simulink model "MirrorSubsystemrepo"  (R2018a)
settings: Solver=VariableStepAuto  StartTime=0.0  StopTime=10.0  RelTol=1e-3
undefined symbols (not defined in the file): sigbuilder_block
libraries: simulink x4
settings Model: Creator=Sushma  LastModifiedBy=training
settings DataIOCC: ReturnWorkspaceOutputs=on
settings SFSimCC: SimUseLocalCustomCode=on
settings RTWCC: RTWUseLocalCustomCode=on

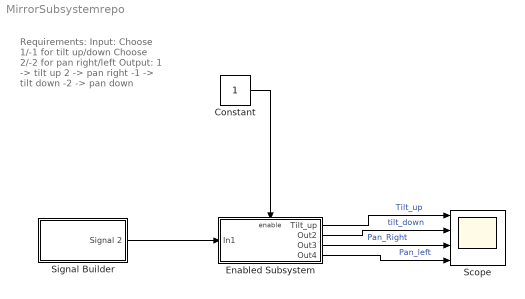
== system MirrorSubsystemrepo ==
  note: Requirements:
      | Input:
      | Choose 1/-1 for tilt up/down
      | Choose 2/-2 for pan right/left
      | Output:
      | 1  ->  tilt up
      | 2  -> pan right
      | -1 -> tilt down
      | -2 -> pan down
  Constant : Constant
  Enabled Subsystem : Subsystem  TreatAsAtomicUnit=on
  Scope : Scope  NumInputPorts=4
  Signal Builder : Subsystem  Tag=STV Subsys  LoadFcn=sigbuilder_block('load');  StartFcn=sigbuilder_block('start');  StopFcn=sigbuilder_block('stop');  ClipboardFcn=sigbuilder_block('clipboard');  mask(Sigbuilder block){tuvar=[0:10]}
      mask help: Simulink:masks:SigbuilderBlock_MD
      mask init:
      | if ~strcmp(get_param(bdroot(gcbh),'SimulationStatus'),'stopped') tuvar = sigbuilder_block('maskInit'); end
      settings: CopyFcn=sigbuilder_block('copy');  DeleteFcn=sigbuilder_block('delete');  ModelCloseFcn=sigbuilder_block('modelClose');  PreSaveFcn=sigbuilder_block('preSave');  PauseFcn=sigbuilder_block('pause');  ContinueFcn=sigbuilder_block('continue');  NameChangeFcn=sigbuilder_block('namechange');  OpenFcn=sigbuilder_block('open',[404 117.5 550.5 362.5 ]);  CloseFcn=sigbuilder_block('close');
      mask Display: plot(0, 0, 100, 100,[2, 2, 32, 32, 2], [68, 8, 8, 68, 68],[32, 2], [38, 38], [32, 19, 2],[53, 60, 44], [32, 17, 17, 2],[16, 16, 31, 31]);txt = getActiveGroup(gcbh);text(2, 100, txt,'verticalAlignment', 'top');
  wires:
  Enabled Subsystem/2(Out2) -> Scope/2  "tilt_down"
  Constant/1 -> Enabled Subsystem/Enable
  Enabled Subsystem/3(Out3) -> Scope/3  "Pan_Right"
  Enabled Subsystem/4(Out4) -> Scope/4  "Pan_left"
  Enabled Subsystem/1(Tilt_up) -> Scope/1  "Tilt_up"
  Signal Builder/1(Signal 2) -> Enabled Subsystem/1(In1)

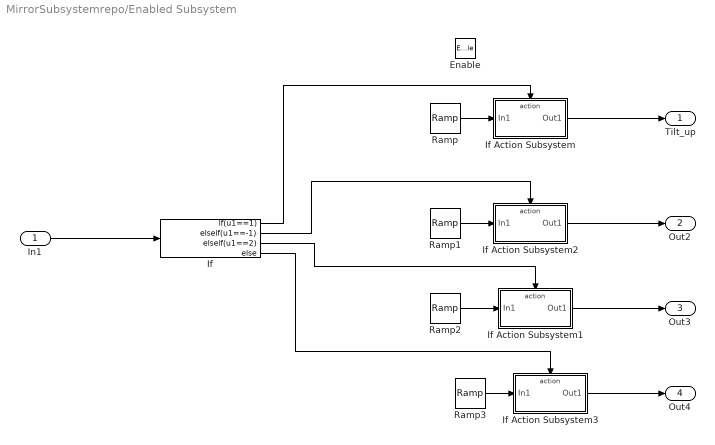
== system MirrorSubsystemrepo/Enabled Subsystem ==
  In1 : Inport
  Enable : EnablePort
  If : If  IfExpression=u1==1  ElseIfExpressions=u1==-1 , u1==2
  If Action Subsystem : Subsystem  TreatAsAtomicUnit=on
  If Action Subsystem1 : Subsystem  TreatAsAtomicUnit=on
  If Action Subsystem2 : Subsystem  TreatAsAtomicUnit=on
  If Action Subsystem3 : Subsystem  TreatAsAtomicUnit=on
  Ramp : simulink/Sources/Ramp  slope=0  start=1  InitialOutput=0
  Ramp1 : simulink/Sources/Ramp  slope=0  start=-1  InitialOutput=0
  Ramp2 : simulink/Sources/Ramp  slope=0  start=0  InitialOutput=2
  Ramp3 : simulink/Sources/Ramp  slope=0  start=0  InitialOutput=-2
  Tilt_up : Outport
  Out2 : Outport  Port=2
  Out3 : Outport  Port=3
  Out4 : Outport  Port=4
  wires:
  If/1 -> If Action Subsystem/Action
  If/2 -> If Action Subsystem2/Action
  If/3 -> If Action Subsystem1/Action
  If/4 -> If Action Subsystem3/Action
  Ramp/1 -> If Action Subsystem/1(In1)
  If Action Subsystem/1(Out1) -> Tilt_up/1
  Ramp1/1 -> If Action Subsystem2/1(In1)
  Ramp2/1 -> If Action Subsystem1/1(In1)
  Ramp3/1 -> If Action Subsystem3/1(In1)
  If Action Subsystem2/1(Out1) -> Out2/1
  If Action Subsystem1/1(Out1) -> Out3/1
  If Action Subsystem3/1(Out1) -> Out4/1
  In1/1 -> If/1

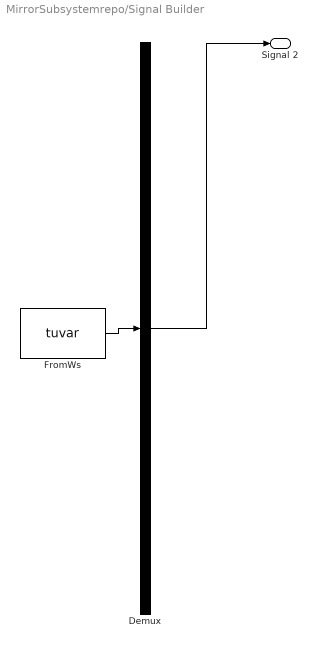
== system MirrorSubsystemrepo/Signal Builder ==
  Demux : Demux  Tag=STV Demux  Outputs=1
      settings: DisplayOption=none
  FromWs : FromWorkspace  Tag=STV FromWs  VariableName=tuvar
      SigBuilderData=|
      | common.afterFinalStr = 'Extrapolate'
      | common.sampleTime = 0
      | dataSet.timeRange = [0 10]
      | dataSet.name = 'Group 1'
      | sbobj.Groups.Name = 'Group 1'
      | sbobj.Groups.Signals.Name = 'Signal 2'
      | sbobj.Groups.Signals.XData = [0 0.5 1 1 1.5 1.5 2 2 2.5 3 3 3.5 3.5 4 4 4.5 4.5 5 5 5.5 5.5 6 6 6.5 6.5 7 7 7.5 8 8.5 8.5 9 9 9.5 9.5 10]
      | sbobj.Groups.Signals.YData = [1 1 1 2 2 -0.98 -0.98 -0.04 -0.04 -0.04 1 1 0 0 2 2 -0.98 -0.98 1.98 1.98 0 0 0.98 0.98 0 0 2 2 2 2 0 0 1.02 1.02 0 0]
  Signal 2 : Outport  Tag=STV Outport
  wires:
  FromWs/1 -> Demux/1
  Demux/1 -> Signal 2/1

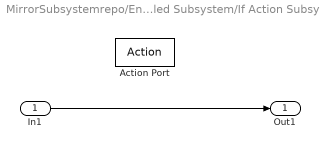
== system MirrorSubsystemrepo/Enabled Subsystem/If Action Subsystem ==
  In1 : Inport
  Action Port : ActionPort
  Out1 : Outport
  wires:
  In1/1 -> Out1/1

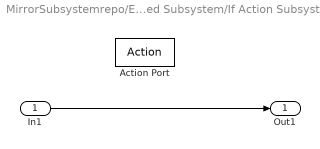
== system MirrorSubsystemrepo/Enabled Subsystem/If Action Subsystem1 ==
  In1 : Inport
  Action Port : ActionPort
  Out1 : Outport
  wires:
  In1/1 -> Out1/1

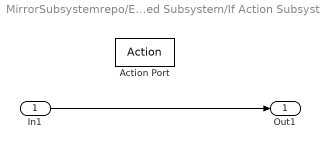
== system MirrorSubsystemrepo/Enabled Subsystem/If Action Subsystem2 ==
  In1 : Inport
  Action Port : ActionPort
  Out1 : Outport
  wires:
  In1/1 -> Out1/1

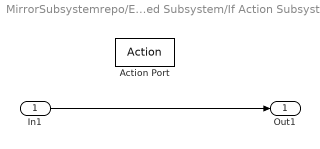
== system MirrorSubsystemrepo/Enabled Subsystem/If Action Subsystem3 ==
  In1 : Inport
  Action Port : ActionPort
  Out1 : Outport
  wires:
  In1/1 -> Out1/1
